simulink model "Diagnostics_R_2024_B_VERSION"  (R2024b)
settings: Solver=VariableStepAuto  StartTime=0.0  StopTime=10.0  RelTol=1e-3
libraries: simulink x1
settings Model: Creator=andym  LastModifiedBy=andym
settings ModelReferenceCC: UpdateModelReferenceTargets=IfOutOfDate
settings ConfigComp: CovBoundaryAbsTol=1.0e-5

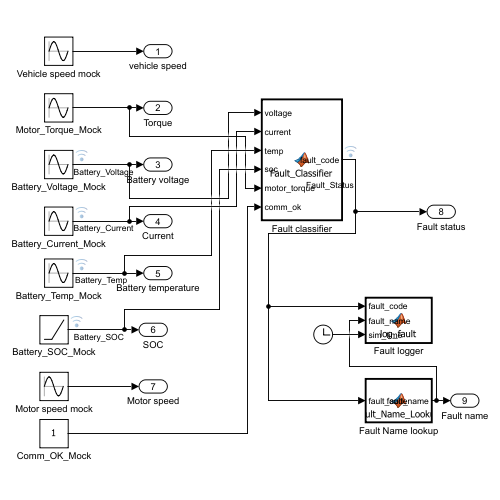
[thumbnail: Simulink's stored preview of the top-level diagram]
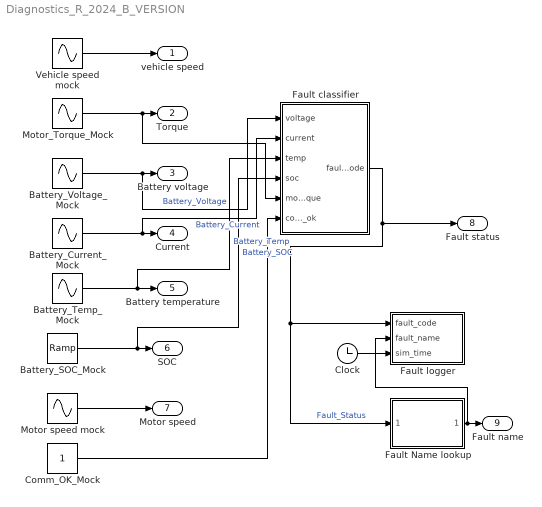
== system Diagnostics_R_2024_B_VERSION ==
  Battery_Current_Mock : Sin  Amplitude=5  Bias=10  Frequency=0.08  SampleTime=0
  Battery_SOC_Mock : simulink/Sources/Ramp  slope=-0.001  start=0  InitialOutput=100
  Battery_Temp_Mock : Sin  Amplitude=3  Bias=30  Frequency=0.02  SampleTime=0
  Battery_Voltage_Mock : Sin  Amplitude=2  Bias=48  Frequency=0.05  SampleTime=0
  Clock : Clock
  Comm_OK_Mock : Constant
  Fault Name lookup : MATLAB Function  TreatAsAtomicUnit=on
  Fault classifier : MATLAB Function  TreatAsAtomicUnit=on
  Fault logger : MATLAB Function  TreatAsAtomicUnit=on
  Motor speed mock : Sin  Amplitude=500  Bias=1500  Frequency=0.1  SampleTime=0
  Motor_Torque_Mock : Sin  Amplitude=10  Bias=20  Frequency=0.12  SampleTime=0
  Vehicle speed mock : Sin  Amplitude=15  Bias=40  Frequency=0.06  SampleTime=0
  vehicle speed : Outport
  Torque : Outport  Port=2
  Battery voltage : Outport  Port=3
  Current : Outport  Port=4
  Battery temperature : Outport  Port=5
  SOC : Outport  Port=6
  Motor speed : Outport  Port=7
  Fault status : Outport  Port=8
  Fault name : Outport  Port=9
  wires:
  Motor speed mock/1 -> Motor speed/1
  Motor_Torque_Mock/1 -> Fault classifier/5(motor_torque), Torque/1
  Battery_SOC_Mock/1 -> SOC/1, Fault classifier/4(soc)  "Battery_SOC"
  Battery_Current_Mock/1 -> Fault classifier/2(current), Current/1  "Battery_Current"
  Battery_Voltage_Mock/1 -> Fault classifier/1(voltage), Battery voltage/1  "Battery_Voltage"
  Vehicle speed mock/1 -> vehicle speed/1
  Battery_Temp_Mock/1 -> Fault classifier/3(temp), Battery temperature/1  "Battery_Temp"
  Fault classifier/1(fault_code) -> Fault Name lookup/1(fault_code), Fault logger/1(fault_code), Fault status/1  "Fault_Status"
  Comm_OK_Mock/1 -> Fault classifier/6(comm_ok)
  Clock/1 -> Fault logger/3(sim_time)
  Fault Name lookup/1(fault_name) -> Fault logger/2(fault_name), Fault name/1

== matlab function Diagnostics_R_2024_B_VERSION/Fault logger ==
  data: fault_code input; fault_name input; sim_time input
function log_fault(fault_code, fault_name, sim_time)

persistent last_code
if isempty(last_code)
    last_code = -1;
end

if fault_code ~= last_code
    fid = fopen('fault_log.csv', 'a');
    if fid ~= -1
        fprintf(fid, '%.3f,%.0f,%s\n', sim_time, fault_code, char(fault_name));
        fclose(fid);
    end
    last_code = fault_code;
end

== matlab function Diagnostics_R_2024_B_VERSION/Fault classifier ==
  data: voltage input; fault_code output; current input; temp input; soc input; motor_torque input; comm_ok input
function fault_code = Fault_Classifier(voltage, current, temp, soc, motor_torque, comm_ok)

persistent state
if isempty(state)
    state = 0; % 0 = Normal
end

if voltage > 58
    state = 1; % F001 Critical - overvoltage
elseif state == 1 && voltage < 55
    state = 0;
end

if temp > 45
    state = 2; % F002 Warning - overtemp
elseif state == 2 && temp < 40
    state = 0;
end

if soc < 5
    state = 3; % F003 Critical - low SOC
elseif state == 3 && soc > 10
    state = 0;
end

if motor_torque > 30
    state = 4; % F004 Warning - overtorque
elseif state == 4 && motor_torque < 25
    state = 0;
end

if comm_ok == 0
    state = 5; % F005 Critical - comms lost
elseif state == 5 && comm_ok == 1
    state = 0;
end

if current > 20
    state = 6; % F006 Critical - overcurrent
elseif state == 6 && current < 17
    state = 0;
end

if voltage < 44
    state = 7; % F007 Critical - undervoltage
elseif state == 7 && voltage > 46
    state = 0;
end

fault_code = state;

== matlab function Diagnostics_R_2024_B_VERSION/Fault Name lookup ==
  data: fault_code input; fault_name output
function fault_name = Fault_Name_Lookup(fault_code)

switch fault_code
    case 0
        raw = 'NORMAL              ';
    case 1
        raw = 'F001 OVERVOLTAGE    ';
    case 2
        raw = 'F002 OVERTEMP       ';
    case 3
        raw = 'F003 LOW SOC        ';
    case 4
        raw = 'F004 OVERTORQUE     ';
    case 5
        raw = 'F005 COMMS LOST     ';
    case 6
        raw = 'F006 OVERCURRENT    ';
    case 7
        raw = 'F007 UNDERVOLTAGE   ';
    otherwise
        raw = 'UNKNOWN FAULT       ';
end

fault_name = uint8(raw);
